simulink model "PC_Quadcopter_Simulation_Hexacopter_health"  (R2022b)
settings: Solver=ode4  StartTime=0.0  StopTime=100  FixedStep=0.01  MaxStep=0.06  RelTol=1e-3
PreLoadFcn:
  | DoB_parameter
model workspace (MAT data in the model file):
  Sig : Simulink.Signal (value not decoded)
values from neighbouring files (symbols this model uses):
  A = [ ... (first row only)    [DoB_parameter.m]
  B = [0 1 0]'    [DoB_parameter.m]
  C = [1 0 0]    [DoB_parameter.m]
  den_Inv_X = conv(num_X,den_Qfilter)    [DoB_parameter.m]
  den_Inv_Y = conv(num_Y, den_Qfilter)    [DoB_parameter.m]
  den_Inv_Z = conv(num_Z, den_Qfilter_Z)    [DoB_parameter.m]
  den_Qfilter = [1 a1/tau a0/tau^2]    [DoB_parameter.m]
  den_Qfilter_Z = [1 a1/tau a0/tau^2]    [DoB_parameter.m]
  I_xx = J(1,1)    [DoB_parameter.m]
  I_yy = J(2,2)    [DoB_parameter.m]
  I_zz = J(3,3)    [DoB_parameter.m]
  IC = block.DialogPrm(2).Data    [quadcopterDynamicsSFunction.m]
  L = [l1 l2 l3]'    [DoB_parameter.m]
  num_Inv_X = conv(den_X,num_Qfilter)    [DoB_parameter.m]
  num_Inv_Y = conv(den_Y, num_Qfilter)    [DoB_parameter.m]
  num_Inv_Z = conv(den_Z, num_Qfilter_Z)    [DoB_parameter.m]
  num_Qfilter = a0/tau^2    (= 100)    [DoB_parameter.m]
  num_Qfilter_Z = a0/tau^2    (= 11.1111111111)    [DoB_parameter.m]
undefined symbols (not defined in the file or in its folder): magnitude, quadModel
libraries: simulink x25, sharedTrackingLibrary x1
(part 2 of 2)

== system PC_Quadcopter_Simulation_Hexacopter_health/Fault Diagnosis/Generate Residual ==
  yMeasured[k] : Inport
  xEstimated[k|k] : Inport  Port=2
  RPM command : Inport  Port=3
  MATLAB Function - Generate Predicted Output : MATLAB Function  TreatAsAtomicUnit=on
  Subtract : Sum  Inputs=+-
  Unit Delay : UnitDelay  InitialCondition=zeros(15,1)  SampleTime=-1  HasFrameUpgradeWarning=on
  Residual : Outport
  wires:
  xEstimated[k|k]/1 -> Unit Delay/1
  Unit Delay/1 -> MATLAB Function - Generate Predicted Output/1(xEstimated)  "xEstimated[k-1|k-1]"
  MATLAB Function - Generate Predicted Output/1(yPredicted) -> Subtract/2  "yPredicted[k|k-1]"
  Subtract/1 -> Residual/1  "e[k]"
  yMeasured[k]/1 -> Subtract/1
  RPM command/1 -> MATLAB Function - Generate Predicted Output/2(u)

== system PC_Quadcopter_Simulation_Hexacopter_health/Hexacopter Dynamics/External Disturbances ==
  note: Note: Torques are in units of N*m, Forces in N
      | Torques are applied to the BODY coordinate system.
      | Forces are applied from the WORLD coordinate system!
      | This can be changed by adjusting the equations within the S-function.
  Bus Creator : BusCreator  Inputs=6
  Bus to Vector : BusToVector
  Constant{1..2,5..6} (4 alike) : Constant  Value=0
  Manual Switch : ManualSwitch
  Manual Switch1 : ManualSwitch
  Step : Step  Time=5  After=0.1  SampleTime=0
  Step2 : Step  Time=10  After=3  SampleTime=0
  "Disturbances " : Outport
  wires:
  Bus to Vector/1 -> "Disturbances "/1
  Bus Creator/1 -> Bus to Vector/1
  Constant6/1 -> Manual Switch1/1, Bus Creator/1  "Tau_bx-axis"
  Constant2/1 -> Bus Creator/3  "Tau_bz-axis"
  Constant1/1 -> Manual Switch/1, Bus Creator/4  "Force_x-axis"
  Constant5/1 -> Bus Creator/6  "Force_z-axis"
  Manual Switch/1 -> Bus Creator/5
  Step2/1 -> Manual Switch/2  "Force_y-axis"
  Manual Switch1/1 -> Bus Creator/2
  Step/1 -> Manual Switch1/2  "Tau_by-axis"

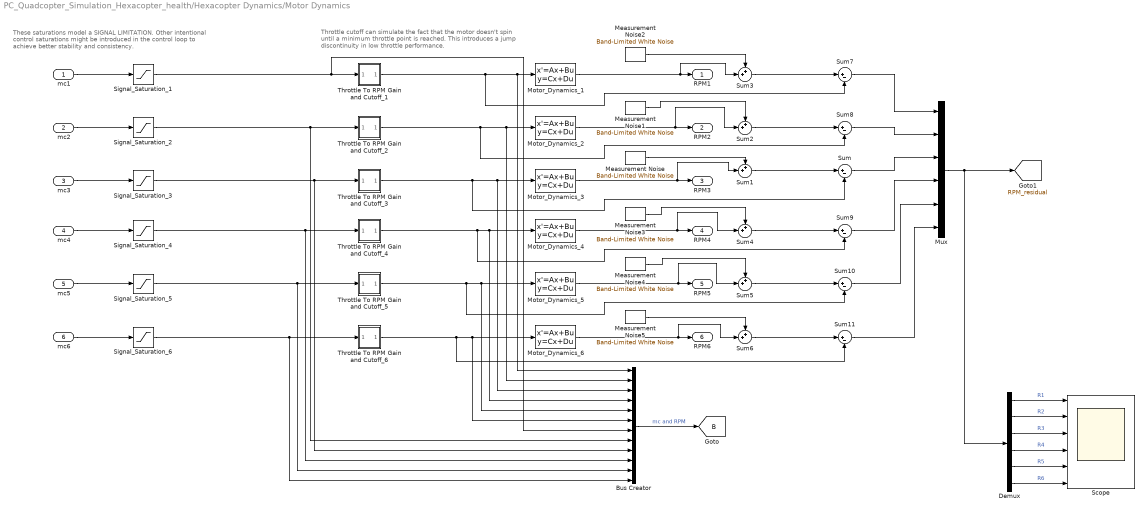
== system PC_Quadcopter_Simulation_Hexacopter_health/Hexacopter Dynamics/Motor Dynamics ==
  note: Throttle cutoff can simulate the fact that the motor doesn't
      | spin until a minimum throttle point is reached. This introduces
      | a jump discontinuity in low throttle performance.
  note: These saturations model a SIGNAL LIMITATION.
      | Other intentional control saturations might be introduced in the
      | control loop to achieve better stability and consistency.
  mc1 : Inport
  mc2 : Inport  Port=2
  mc3 : Inport  Port=3
  mc4 : Inport  Port=4
  mc5 : Inport  Port=5
  mc6 : Inport  Port=6
  Bus Creator : BusCreator  Inputs=12
  Demux : Demux  Outputs=6
  Measurement Noise{,1..5} (6 alike) : simulink/Sources/Band-Limited White Noise  Cov=10^2  Ts=0.02  seed=[23342]
  Motor_Dynamics_1 : StateSpace  A=-1/quadModel.T  C=1/quadModel.T  D=0  InitialCondition=IC.w1*quadModel.T
  Motor_Dynamics_2 : StateSpace  A=-1/quadModel.T  C=1/quadModel.T  D=0  InitialCondition=IC.w2*quadModel.T
  Motor_Dynamics_3 : StateSpace  A=-1/quadModel.T  C=1/quadModel.T  D=0  InitialCondition=IC.w3*quadModel.T
  Motor_Dynamics_4 : StateSpace  A=-1/quadModel.T  C=1/quadModel.T  D=0  InitialCondition=IC.w4*quadModel.T
  Motor_Dynamics_5 : StateSpace  A=-1/quadModel.T  C=1/quadModel.T  D=0  InitialCondition=IC.w4*quadModel.T
  Motor_Dynamics_6 : StateSpace  A=-1/quadModel.T  C=1/quadModel.T  D=0  InitialCondition=IC.w4*quadModel.T
  Mux : Mux  Inputs=6
  Scope : Scope  NumInputPorts=6
  Signal_Saturation_{1..6} (6 alike) : Saturate  UpperLimit=100  LowerLimit=0
  Sum{,7..11} (6 alike) : Sum  Inputs=|+-
  Sum{1..6} (6 alike) : Sum  Inputs=++|
  Throttle To RPM Gain and Cutoff_1 : Subsystem
  Throttle To RPM Gain and Cutoff_2 : Subsystem
  Throttle To RPM Gain and Cutoff_3 : Subsystem
  Throttle To RPM Gain and Cutoff_4 : Subsystem
  Throttle To RPM Gain and Cutoff_5 : Subsystem
  Throttle To RPM Gain and Cutoff_6 : Subsystem
  RPM1 : Outport
  RPM2 : Outport  Port=2
  RPM3 : Outport  Port=3
  RPM4 : Outport  Port=4
  RPM5 : Outport  Port=5
  RPM6 : Outport  Port=6
  tag scope: B=global, RPM_residual=global
  wires:
  mc1/1 -> Signal_Saturation_1/1
  mc4/1 -> Signal_Saturation_4/1
  mc2/1 -> Signal_Saturation_2/1
  mc3/1 -> Signal_Saturation_3/1
  Signal_Saturation_1/1 -> Bus Creator/7, Throttle To RPM Gain and Cutoff_1/1(In5)
  Signal_Saturation_2/1 -> Throttle To RPM Gain and Cutoff_2/1(In5), Bus Creator/8
  Signal_Saturation_3/1 -> Bus Creator/9, Throttle To RPM Gain and Cutoff_3/1(In5)
  Signal_Saturation_4/1 -> Bus Creator/10, Throttle To RPM Gain and Cutoff_4/1(In5)
  Throttle To RPM Gain and Cutoff_1/1(Out5) -> Sum7/2, Bus Creator/1, Motor_Dynamics_1/1
  Throttle To RPM Gain and Cutoff_2/1(Out5) -> Sum8/2, Motor_Dynamics_2/1, Bus Creator/2
  Throttle To RPM Gain and Cutoff_3/1(Out5) -> Sum/2, Motor_Dynamics_3/1, Bus Creator/3
  Throttle To RPM Gain and Cutoff_4/1(Out5) -> Sum9/2, Motor_Dynamics_4/1, Bus Creator/4
  Motor_Dynamics_1/1 -> Sum3/2, RPM1/1
  Motor_Dynamics_2/1 -> Sum2/2, RPM2/1
  Motor_Dynamics_3/1 -> Sum1/2, RPM3/1
  Motor_Dynamics_4/1 -> Sum4/2, RPM4/1
  Bus Creator/1 -> [B]  "mc and RPM"
  Motor_Dynamics_5/1 -> Sum5/2, RPM5/1
  mc5/1 -> Signal_Saturation_5/1
  Signal_Saturation_5/1 -> Bus Creator/11, Throttle To RPM Gain and Cutoff_5/1(In5)
  Throttle To RPM Gain and Cutoff_5/1(Out5) -> Sum10/2, Motor_Dynamics_5/1, Bus Creator/5
  Motor_Dynamics_6/1 -> Sum6/2, RPM6/1
  mc6/1 -> Signal_Saturation_6/1
  Signal_Saturation_6/1 -> Bus Creator/12, Throttle To RPM Gain and Cutoff_6/1(In5)
  Throttle To RPM Gain and Cutoff_6/1(Out5) -> Sum11/2, Motor_Dynamics_6/1, Bus Creator/6
  Mux/1 -> Demux/1, [RPM_residual]
  Measurement Noise/1 -> Sum1/1
  Sum1/1 -> Sum/1
  Measurement Noise5/1 -> Sum6/1
  Measurement Noise4/1 -> Sum5/1
  Measurement Noise3/1 -> Sum4/1
  Measurement Noise1/1 -> Sum2/1
  Measurement Noise2/1 -> Sum3/1
  Sum2/1 -> Sum8/1
  Sum3/1 -> Sum7/1
  Sum4/1 -> Sum9/1
  Sum5/1 -> Sum10/1
  Sum6/1 -> Sum11/1
  Sum7/1 -> Mux/1
  Sum8/1 -> Mux/2
  Sum/1 -> Mux/3
  Sum9/1 -> Mux/4
  Sum10/1 -> Mux/5
  Sum11/1 -> Mux/6
  Demux/6 -> Scope/6  "R6"
  Demux/5 -> Scope/5  "R5"
  Demux/4 -> Scope/4  "R4"
  Demux/3 -> Scope/3  "R3"
  Demux/2 -> Scope/2  "R2"
  Demux/1 -> Scope/1  "R1"

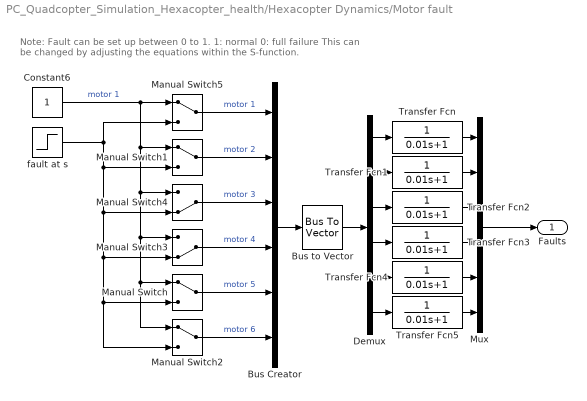
== system PC_Quadcopter_Simulation_Hexacopter_health/Hexacopter Dynamics/Motor fault ==
  note: Note: Fault can be set up between 0 to 1.
      | 1: normal
      | 0: full failure
      | This can be changed by adjusting the equations within the S-function.
  Bus Creator : BusCreator  Inputs=6
  Bus to Vector : BusToVector
  Constant6 : Constant
  Demux : Demux  Outputs=6
  Manual Switch{,1..2,5} (4 alike) : ManualSwitch
  Manual Switch3 : ManualSwitch  CurrentSetting=0
  Manual Switch4 : ManualSwitch  CurrentSetting=0
  Mux : Mux  Inputs=6
  Transfer Fcn{,1..5} (6 alike) : TransferFcn  Numerator=1  Denominator=[0.01 1]
  fault at s : Step  Time=85  Before=1  After=0  SampleTime=0
  Faults : Outport
  wires:
  Manual Switch1/1 -> Bus Creator/2  "motor 2"
  Manual Switch/1 -> Bus Creator/5  "motor 5"
  Bus Creator/1 -> Bus to Vector/1
  Manual Switch2/1 -> Bus Creator/6  "motor 6"
  Manual Switch3/1 -> Bus Creator/4  "motor 4"
  Demux/1 -> Transfer Fcn/1
  Demux/2 -> Transfer Fcn1/1
  Demux/3 -> Transfer Fcn2/1
  Demux/6 -> Transfer Fcn5/1
  Demux/5 -> Transfer Fcn4/1
  Demux/4 -> Transfer Fcn3/1
  Transfer Fcn/1 -> Mux/1
  Transfer Fcn1/1 -> Mux/2
  Transfer Fcn2/1 -> Mux/3
  Transfer Fcn4/1 -> Mux/5
  Transfer Fcn5/1 -> Mux/6
  Transfer Fcn3/1 -> Mux/4
  Manual Switch4/1 -> Bus Creator/3  "motor 3"
  Constant6/1 -> Manual Switch5/1, Manual Switch2/1, Manual Switch/1, Manual Switch3/1, Manual Switch4/1, Manual Switch1/1  "motor 1"
  Manual Switch5/1 -> Bus Creator/1  "motor 1"
  fault at s/1 -> Manual Switch2/2, Manual Switch/2, Manual Switch3/2, Manual Switch4/2, Manual Switch1/2, Manual Switch5/2
  Bus to Vector/1 -> Demux/1
  Mux/1 -> Faults/1

== system PC_Quadcopter_Simulation_Hexacopter_health/Hexacopter Dynamics/a_x, a_y, a_z ==
  p : Inport
  q : Inport  Port=2
  r : Inport  Port=3
  U : Inport  Port=4
  V : Inport  Port=5
  W : Inport  Port=6
  Phi : Inport  Port=7
  Theta : Inport  Port=8
  Subsystem : Subsystem
  Subsystem1 : Subsystem
  Subsystem2 : Subsystem
  a_x : Outport
  a_y : Outport  Port=2
  a_z : Outport  Port=3
  wires:
  Subsystem/1(a_x) -> a_x/1
  Subsystem1/1(a_y) -> a_y/1
  Subsystem2/1(a_z) -> a_z/1
  q/1 -> Subsystem2/2(q), Subsystem/1(q)
  r/1 -> Subsystem/2(r), Subsystem1/2(r)
  U/1 -> Subsystem2/3(U), Subsystem1/3(U), Subsystem/3(U)
  V/1 -> Subsystem2/4(V), Subsystem/4(V), Subsystem1/4(V)
  W/1 -> Subsystem2/5(W), Subsystem/5(W), Subsystem1/5(W)
  Theta/1 -> Subsystem2/7(Theta), Subsystem1/7(Theta), Subsystem/6(Theta)
  p/1 -> Subsystem2/1(p), Subsystem1/1(p)
  Phi/1 -> Subsystem2/6(Phi), Subsystem1/6(Phi)

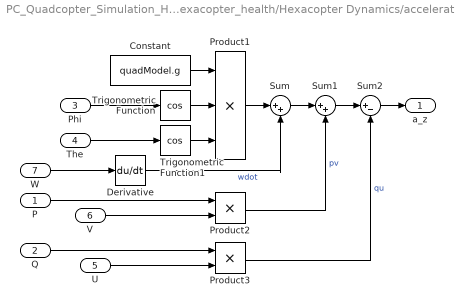
== system PC_Quadcopter_Simulation_Hexacopter_health/Hexacopter Dynamics/acceleration ==
  P : Inport
  Q : Inport  Port=2
  Phi : Inport  Port=3
  The : Inport  Port=4
  U : Inport  Port=5
  V : Inport  Port=6
  W : Inport  Port=7
  Constant : Constant  Value=quadModel.g
  Derivative : Derivative
  Product1 : Product  Inputs=3
  Product2 : Product
  Product3 : Product
  Sum : Sum  Inputs=|++
  Sum1 : Sum  Inputs=|++
  Sum2 : Sum  Inputs=|+-
  Trigonometric Function : Trigonometry  Operator=cos
  Trigonometric Function1 : Trigonometry  Operator=cos
  a_z : Outport
  wires:
  Trigonometric Function/1 -> Product1/2
  Sum/1 -> Sum1/1
  Derivative/1 -> Sum/2  "wdot"
  Trigonometric Function1/1 -> Product1/3
  W/1 -> Derivative/1
  Constant/1 -> Product1/1
  Sum1/1 -> Sum2/1
  Phi/1 -> Trigonometric Function/1
  V/1 -> Product2/2
  P/1 -> Product2/1
  U/1 -> Product3/2
  Sum2/1 -> a_z/1
  The/1 -> Trigonometric Function1/1
  Q/1 -> Product3/1
  Product2/1 -> Sum1/2  "pv"
  Product3/1 -> Sum2/2  "qu"
  Product1/1 -> Sum/1

== system PC_Quadcopter_Simulation_Hexacopter_health/LESO/Linear Extended-State Observer ==
  y : Inport
  u : Inport  Port=2
  Add3 : Sum  Inputs=+++
  Demux : Demux  Outputs=3
  Integrator : Integrator
  Terminator : Terminator
  theta1 : Gain  Gain=B  Multiplication=Matrix(K*u)
  theta10 : Gain  Gain=L  Multiplication=Matrix(K*u)
  theta2 : Gain  Gain=A-L*C  Multiplication=Matrix(K*u)
  x2_hat : Outport
  x3_hat (F) : Outport  Port=2
  wires:
  theta1/1 -> Add3/2
  theta10/1 -> Add3/1
  y/1 -> theta10/1
  u/1 -> theta1/1
  Add3/1 -> Integrator/1
  theta2/1 -> Add3/3
  Demux/3 -> x3_hat (F)/1
  Demux/2 -> x2_hat/1
  Integrator/1 -> theta2/1, Demux/1
  Demux/1 -> Terminator/1

== system PC_Quadcopter_Simulation_Hexacopter_health/LESO/Linear Extended-State Observer1 ==
  y : Inport
  u : Inport  Port=2
  Add3 : Sum  Commented=on  Inputs=+++
  Demux : Demux  Commented=on  Outputs=3
  Integrator : Integrator  Commented=on
  Terminator : Terminator  Commented=on
  theta1 : Gain  Commented=on  Gain=B  Multiplication=Matrix(K*u)
  theta10 : Gain  Commented=on  Gain=L  Multiplication=Matrix(K*u)
  theta2 : Gain  Commented=on  Gain=A-L*C  Multiplication=Matrix(K*u)
  x2_hat : Outport
  x3_hat (F) : Outport  Port=2
  wires:
  Demux/1 -> Terminator/1
  Integrator/1 -> Demux/1, theta2/1
  Demux/2 -> x2_hat/1
  Demux/3 -> x3_hat (F)/1
  theta2/1 -> Add3/3
  Add3/1 -> Integrator/1
  u/1 -> theta1/1
  y/1 -> theta10/1
  theta10/1 -> Add3/1
  theta1/1 -> Add3/2

== system PC_Quadcopter_Simulation_Hexacopter_health/LESO/Linear Extended-State Observer2 ==
  y : Inport
  u : Inport  Port=2
  Add3 : Sum  Inputs=+++
  Demux : Demux  Outputs=3
  Integrator : Integrator
  Terminator : Terminator
  theta1 : Gain  Gain=B  Multiplication=Matrix(K*u)
  theta10 : Gain  Gain=L  Multiplication=Matrix(K*u)
  theta2 : Gain  Gain=A-L*C  Multiplication=Matrix(K*u)
  x2_hat : Outport
  x3_hat (F) : Outport  Port=2
  wires:
  theta1/1 -> Add3/2
  theta10/1 -> Add3/1
  y/1 -> theta10/1
  u/1 -> theta1/1
  Add3/1 -> Integrator/1
  theta2/1 -> Add3/3
  Demux/3 -> x3_hat (F)/1
  Demux/2 -> x2_hat/1
  Integrator/1 -> theta2/1, Demux/1
  Demux/1 -> Terminator/1

== system PC_Quadcopter_Simulation_Hexacopter_health/Position Controller/Altitude (Z) Control ==
  note: Improve to use rotation matrix and euler angles...
      | maybe with saturation?
  note: ez
  Desired Z : Inport
  Bus Selector : BusSelector  OutputSignals=Alt_Cmd
  Gravity Offset (Level Flight) : Constant  Value=GOffset
  Integrator Limited : Integrator  LimitOutput=on  UpperSaturationLimit=USat  LowerSaturationLimit=LSat
  Kiz : Gain  Gain=Kiz
  Kpz : Gain  Gain=Kpz
  Sum : Sum  Inputs=|+|
  Sum2 : Sum  Inputs=+++
  Alt. (Z) Correction : Outport
  wires:
  Gravity Offset (Level Flight)/1 -> Sum2/1
  Desired Z/1 -> Bus Selector/1
  Sum2/1 -> Alt. (Z) Correction/1
  Kpz/1 -> Sum2/2  "P Corr"
  Sum/1 -> Integrator Limited/1, Kpz/1  "Error"
  Kiz/1 -> Sum2/3  "I Corr"
  Integrator Limited/1 -> Kiz/1
  Bus Selector/1 -> Sum/1  "<Alt_Cmd>"

== system PC_Quadcopter_Simulation_Hexacopter_health/Position Controller/Error Rotations ==
  X_cmd : Inport
  Y_cmd : Inport  Port=2
  X : Inport  Port=3
  Y : Inport  Port=4
  Psi : Inport  Port=5
  Product{,1..3} (4 alike) : Product
  Sum : Sum  Inputs=|+-
  Sum1 : Sum  Inputs=|+-
  Sum2 : Sum  Inputs=|++
  Sum4 : Sum  Inputs=|+-
  Trigonometric Functions : Trigonometry  Operator=sincos
  X Error in body Frame : Outport
  Y Error in Body Frame : Outport  Port=2
  wires:
  Sum4/1 -> Y Error in Body Frame/1  "Yerr*cos(psi)-Xerr*sin(psi)"
  Product3/1 -> Sum4/2  "Xerr*sin(psi)"
  Sum1/1 -> Product2/1, Product1/1  "Y Error"
  Trigonometric Functions/1 -> Product2/2, Product3/2  "sin(psi)"
  Sum2/1 -> X Error in body Frame/1  "Xerr*cos(psi)+Yerr*sin(psi)"
  Y_cmd/1 -> Sum1/1
  X_cmd/1 -> Sum/1
  X/1 -> Sum/2
  Y/1 -> Sum1/2
  Sum/1 -> Product3/1, Product/1  "X Error"
  Trigonometric Functions/2 -> Product/2, Product1/2  "cos(psi)"
  Product/1 -> Sum2/1  "Xerr*cos(psi)"
  Product2/1 -> Sum2/2  "Yerr*sin(psi)"
  Product1/1 -> Sum4/1  "Yerr*cos(psi)"
  Psi/1 -> Trigonometric Functions/1

== system PC_Quadcopter_Simulation_Hexacopter_health/Position Controller/Error Rotations1 ==
  X_cmd : Inport
  Y_cmd : Inport  Port=2
  Constant : Constant  Value=0
  Product{,1..3} (4 alike) : Product
  Sum2 : Sum  Inputs=|++
  Sum4 : Sum  Inputs=|+-
  Trigonometric Functions : Trigonometry  Operator=sincos
  X Error in body Frame : Outport
  Y Error in Body Frame : Outport  Port=2
  wires:
  Constant/1 -> Trigonometric Functions/1
  Product1/1 -> Sum4/1  "Yerr*cos(psi)"
  Product2/1 -> Sum2/2  "Yerr*sin(psi)"
  Product/1 -> Sum2/1  "Xerr*cos(psi)"
  Trigonometric Functions/2 -> Product1/2, Product/2  "cos(psi)"
  X_cmd/1 -> Product/1, Product3/1  "X Error"
  Sum2/1 -> X Error in body Frame/1  "Xerr*cos(psi)+Yerr*sin(psi)"
  Trigonometric Functions/1 -> Product3/2, Product2/2  "sin(psi)"
  Y_cmd/1 -> Product1/1, Product2/1  "Y Error"
  Product3/1 -> Sum4/2  "Xerr*sin(psi)"
  Sum4/1 -> Y Error in Body Frame/1  "Yerr*cos(psi)-Xerr*sin(psi)"

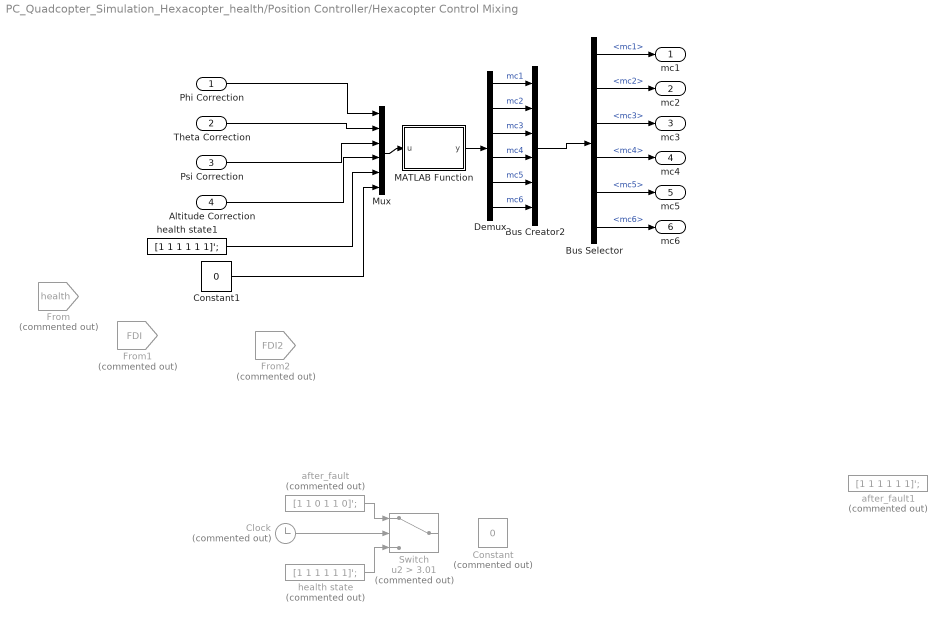
== system PC_Quadcopter_Simulation_Hexacopter_health/Position Controller/Hexacopter Control Mixing ==
  Phi Correction : Inport
  Theta Correction : Inport  Port=2
  Psi Correction : Inport  Port=3
  Altitude Correction : Inport  Port=4
  Bus Creator2 : BusCreator  Inputs=6
  Bus Selector : BusSelector  OutputSignals=mc1,mc2,mc3,mc4,mc5,mc6
  Clock : Clock  Commented=on
  Constant : Constant  Commented=on  Value=0
  Constant1 : Constant  Value=0
  Demux : Demux  Outputs=6
  From : From  Commented=on  GotoTag=health  TagVisibility=global
  From1 : From  Commented=on  GotoTag=FDI  TagVisibility=global
  From2 : From  Commented=on  GotoTag=FDI2  TagVisibility=global
  MATLAB Function : MATLAB Function  TreatAsAtomicUnit=on
  Mux : Mux  Inputs=6
  Switch : Switch  Commented=on  Criteria=u2 > Threshold  Threshold=3.01  SaturateOnIntegerOverflow=off  InputSameDT=off
  after_fault : Constant  Commented=on  Value=[1 1 0 1 1 0]';
  after_fault1 : Constant  Commented=on  Value=[1 1 1 1 1 1]';
  health state : Constant  Commented=on  Value=[1 1 1 1 1 1]';
  health state1 : Constant  Value=[1 1 1 1 1 1]';
  mc1 : Outport
  mc2 : Outport  Port=2
  mc3 : Outport  Port=3
  mc4 : Outport  Port=4
  mc5 : Outport  Port=5
  mc6 : Outport  Port=6
  wires:
  Phi Correction/1 -> Mux/1
  Theta Correction/1 -> Mux/2
  Psi Correction/1 -> Mux/3
  Altitude Correction/1 -> Mux/4
  Bus Selector/1 -> mc1/1  "<mc1>"
  Bus Selector/2 -> mc2/1  "<mc2>"
  Bus Selector/3 -> mc3/1  "<mc3>"
  Bus Selector/4 -> mc4/1  "<mc4>"
  Bus Selector/5 -> mc5/1  "<mc5>"
  Bus Selector/6 -> mc6/1  "<mc6>"
  Mux/1 -> MATLAB Function/1(u)
  MATLAB Function/1(y) -> Demux/1
  Demux/6 -> Bus Creator2/6  "mc6"
  Demux/3 -> Bus Creator2/3  "mc3"
  Demux/4 -> Bus Creator2/4  "mc4"
  Demux/1 -> Bus Creator2/1  "mc1"
  Demux/5 -> Bus Creator2/5  "mc5"
  Demux/2 -> Bus Creator2/2  "mc2"
  Bus Creator2/1 -> Bus Selector/1
  Constant1/1 -> Mux/6
  health state1/1 -> Mux/5
  health state/1 -> Switch/3
  after_fault/1 -> Switch/1
  Clock/1 -> Switch/2

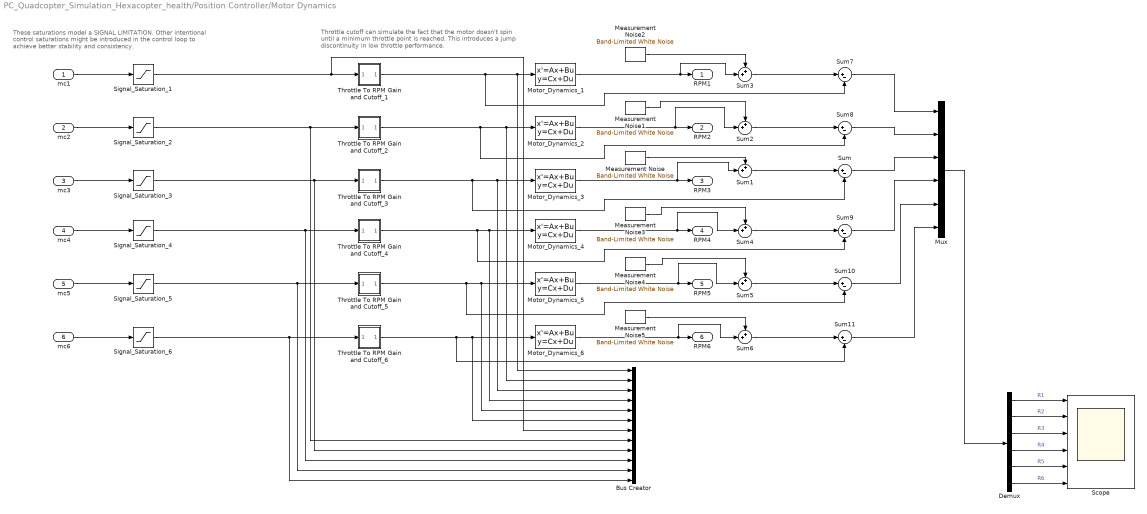
== system PC_Quadcopter_Simulation_Hexacopter_health/Position Controller/Motor Dynamics ==
  note: Throttle cutoff can simulate the fact that the motor doesn't
      | spin until a minimum throttle point is reached. This introduces
      | a jump discontinuity in low throttle performance.
  note: These saturations model a SIGNAL LIMITATION.
      | Other intentional control saturations might be introduced in the
      | control loop to achieve better stability and consistency.
  mc1 : Inport
  mc2 : Inport  Port=2
  mc3 : Inport  Port=3
  mc4 : Inport  Port=4
  mc5 : Inport  Port=5
  mc6 : Inport  Port=6
  Bus Creator : BusCreator  Inputs=12
  Demux : Demux  Outputs=6
  Measurement Noise{,1..5} (6 alike) : simulink/Sources/Band-Limited White Noise  Cov=10^2  Ts=0.02  seed=[23342]
  Motor_Dynamics_1 : StateSpace  A=-1/quadModel.T  C=1/quadModel.T  D=0  InitialCondition=IC.w1*quadModel.T
  Motor_Dynamics_2 : StateSpace  A=-1/quadModel.T  C=1/quadModel.T  D=0  InitialCondition=IC.w2*quadModel.T
  Motor_Dynamics_3 : StateSpace  A=-1/quadModel.T  C=1/quadModel.T  D=0  InitialCondition=IC.w3*quadModel.T
  Motor_Dynamics_4 : StateSpace  A=-1/quadModel.T  C=1/quadModel.T  D=0  InitialCondition=IC.w4*quadModel.T
  Motor_Dynamics_5 : StateSpace  A=-1/quadModel.T  C=1/quadModel.T  D=0  InitialCondition=IC.w4*quadModel.T
  Motor_Dynamics_6 : StateSpace  A=-1/quadModel.T  C=1/quadModel.T  D=0  InitialCondition=IC.w4*quadModel.T
  Mux : Mux  Inputs=6
  Scope : Scope  NumInputPorts=6
  Signal_Saturation_{1..6} (6 alike) : Saturate  UpperLimit=100  LowerLimit=0
  Sum{,7..11} (6 alike) : Sum  Inputs=|+-
  Sum{1..6} (6 alike) : Sum  Inputs=++|
  Throttle To RPM Gain and Cutoff_1 : Subsystem
  Throttle To RPM Gain and Cutoff_2 : Subsystem
  Throttle To RPM Gain and Cutoff_3 : Subsystem
  Throttle To RPM Gain and Cutoff_4 : Subsystem
  Throttle To RPM Gain and Cutoff_5 : Subsystem
  Throttle To RPM Gain and Cutoff_6 : Subsystem
  RPM1 : Outport
  RPM2 : Outport  Port=2
  RPM3 : Outport  Port=3
  RPM4 : Outport  Port=4
  RPM5 : Outport  Port=5
  RPM6 : Outport  Port=6
  wires:
  mc1/1 -> Signal_Saturation_1/1
  mc4/1 -> Signal_Saturation_4/1
  mc2/1 -> Signal_Saturation_2/1
  mc3/1 -> Signal_Saturation_3/1
  Signal_Saturation_1/1 -> Bus Creator/7, Throttle To RPM Gain and Cutoff_1/1(In5)
  Signal_Saturation_2/1 -> Throttle To RPM Gain and Cutoff_2/1(In5), Bus Creator/8
  Signal_Saturation_3/1 -> Bus Creator/9, Throttle To RPM Gain and Cutoff_3/1(In5)
  Signal_Saturation_4/1 -> Bus Creator/10, Throttle To RPM Gain and Cutoff_4/1(In5)
  Throttle To RPM Gain and Cutoff_1/1(Out5) -> Sum7/2, Bus Creator/1, Motor_Dynamics_1/1
  Throttle To RPM Gain and Cutoff_2/1(Out5) -> Sum8/2, Motor_Dynamics_2/1, Bus Creator/2
  Throttle To RPM Gain and Cutoff_3/1(Out5) -> Sum/2, Motor_Dynamics_3/1, Bus Creator/3
  Throttle To RPM Gain and Cutoff_4/1(Out5) -> Sum9/2, Motor_Dynamics_4/1, Bus Creator/4
  Motor_Dynamics_1/1 -> Sum3/2, RPM1/1
  Motor_Dynamics_2/1 -> Sum2/2, RPM2/1
  Motor_Dynamics_3/1 -> Sum1/2, RPM3/1
  Motor_Dynamics_4/1 -> Sum4/2, RPM4/1
  Motor_Dynamics_5/1 -> Sum5/2, RPM5/1
  mc5/1 -> Signal_Saturation_5/1
  Signal_Saturation_5/1 -> Bus Creator/11, Throttle To RPM Gain and Cutoff_5/1(In5)
  Throttle To RPM Gain and Cutoff_5/1(Out5) -> Sum10/2, Motor_Dynamics_5/1, Bus Creator/5
  Motor_Dynamics_6/1 -> Sum6/2, RPM6/1
  mc6/1 -> Signal_Saturation_6/1
  Signal_Saturation_6/1 -> Bus Creator/12, Throttle To RPM Gain and Cutoff_6/1(In5)
  Throttle To RPM Gain and Cutoff_6/1(Out5) -> Sum11/2, Motor_Dynamics_6/1, Bus Creator/6
  Mux/1 -> Demux/1
  Measurement Noise/1 -> Sum1/1
  Sum1/1 -> Sum/1
  Measurement Noise5/1 -> Sum6/1
  Measurement Noise4/1 -> Sum5/1
  Measurement Noise3/1 -> Sum4/1
  Measurement Noise1/1 -> Sum2/1
  Measurement Noise2/1 -> Sum3/1
  Sum2/1 -> Sum8/1
  Sum3/1 -> Sum7/1
  Sum4/1 -> Sum9/1
  Sum5/1 -> Sum10/1
  Sum6/1 -> Sum11/1
  Sum7/1 -> Mux/1
  Sum8/1 -> Mux/2
  Sum/1 -> Mux/3
  Sum9/1 -> Mux/4
  Sum10/1 -> Mux/5
  Sum11/1 -> Mux/6
  Demux/6 -> Scope/6  "R6"
  Demux/5 -> Scope/5  "R5"
  Demux/4 -> Scope/4  "R4"
  Demux/3 -> Scope/3  "R3"
  Demux/2 -> Scope/2  "R2"
  Demux/1 -> Scope/1  "R1"

== system PC_Quadcopter_Simulation_Hexacopter_health/Position Controller/Phi Command Control ==
  note: -1 Gain is required because a "negative"
      | angle of Phi induces a positive velocity
      | in the body frame y direction!
  Desired Yb Velocity : Inport
  Yb Velocity : Inport  Port=2
  Attitude Limits_Phi : Saturate  UpperLimit=ASat  LowerLimit=-ASat
  Gain : Gain  Gain=-1
  Kdp : Gain  Gain=Kd
  Kpp : Gain  Gain=Kp
  Sum3 : Sum  Inputs=|+-
  Sum6 : Sum  Inputs=|+-
  V Derivative : Derivative
  Phi_cmd : Outport
  wires:
  V Derivative/1 -> Kdp/1
  Attitude Limits_Phi/1 -> Phi_cmd/1  "Phi_cmd"
  Sum6/1 -> Gain/1
  Kpp/1 -> Sum6/1
  Sum3/1 -> Kpp/1  "Velocity Error"
  Yb Velocity/1 -> V Derivative/1, Sum3/2
  Desired Yb Velocity/1 -> Sum3/1
  Gain/1 -> Attitude Limits_Phi/1
  Kdp/1 -> Sum6/2

== system PC_Quadcopter_Simulation_Hexacopter_health/Position Controller/Phi Command Control1 ==
  note: -1 Gain is required because a "negative"
      | angle of Phi induces a positive velocity
      | in the body frame y direction!
  Desired Yb Velocity : Inport
  Attitude Limits_Phi : Saturate  UpperLimit=ASat  LowerLimit=-ASat
  Gain : Gain  Gain=-1
  Kpp : Gain  Gain=Kp
  Phi_cmd : Outport
  wires:
  Gain/1 -> Attitude Limits_Phi/1
  Desired Yb Velocity/1 -> Kpp/1  "Velocity Error"
  Kpp/1 -> Gain/1
  Attitude Limits_Phi/1 -> Phi_cmd/1  "Phi_cmd"

== system PC_Quadcopter_Simulation_Hexacopter_health/Position Controller/Pitch (Theta) Control ==
  Attitude Command : Inport
  Bus Selector : BusSelector  OutputSignals=The_cmd
  Integrator Limited : Integrator  LimitOutput=on  UpperSaturationLimit=USat  LowerSaturationLimit=LSat
  Kit : Gain  Gain=Kit
  Kpt : Gain  Gain=Kpt
  Sum1 : Sum  Inputs=++|
  Theta Correction : Outport
  wires:
  Attitude Command/1 -> Bus Selector/1
  Sum1/1 -> Theta Correction/1
  Kpt/1 -> Sum1/1  "P Corr"
  Kit/1 -> Sum1/2  "I Corr"
  Integrator Limited/1 -> Kit/1
  Bus Selector/1 -> Integrator Limited/1, Kpt/1  "<The_cmd>"

== system PC_Quadcopter_Simulation_Hexacopter_health/Position Controller/Roll (Phi) Control  ==
  "Attitude Command " : Inport
  Bus Selector : BusSelector  OutputSignals=Phi_cmd
  Integrator Limited : Integrator  LimitOutput=on  UpperSaturationLimit=USat  LowerSaturationLimit=LSat
  Kip : Gain  Gain=Kip
  Kpp : Gain  Gain=Kpp
  Sum1 : Sum  Inputs=++|
  Phi Correction : Outport
  wires:
  Sum1/1 -> Phi Correction/1
  Kpp/1 -> Sum1/1  "P Corr"
  Kip/1 -> Sum1/2  "I Corr"
  Integrator Limited/1 -> Kip/1
  "Attitude Command "/1 -> Bus Selector/1
  Bus Selector/1 -> Integrator Limited/1, Kpp/1  "<Phi_cmd>"

== system PC_Quadcopter_Simulation_Hexacopter_health/Position Controller/Theta Command Control ==
  Desired Xb Velocity : Inport
  Xb Velocity : Inport  Port=2
  Attitude Limits_Theta : Saturate  UpperLimit=ASat  LowerLimit=-ASat
  Kdt : Gain  Gain=Kd
  Kpt : Gain  Gain=Kp
  Sum3 : Sum  Inputs=|+-
  Sum6 : Sum  Inputs=|+-
  U Derivative : Derivative
  The_cmd : Outport
  wires:
  Kdt/1 -> Sum6/2
  U Derivative/1 -> Kdt/1
  Attitude Limits_Theta/1 -> The_cmd/1  "The_cmd"
  Sum6/1 -> Attitude Limits_Theta/1
  Kpt/1 -> Sum6/1
  Sum3/1 -> Kpt/1  "Velocity Error"
  Xb Velocity/1 -> U Derivative/1, Sum3/2
  Desired Xb Velocity/1 -> Sum3/1

== system PC_Quadcopter_Simulation_Hexacopter_health/Position Controller/Theta Command Control1 ==
  Desired Xb Velocity : Inport
  Attitude Limits_Theta : Saturate  UpperLimit=ASat  LowerLimit=-ASat
  Kpt : Gain  Gain=Kp
  The_cmd : Outport
  wires:
  Desired Xb Velocity/1 -> Kpt/1  "Velocity Error"
  Kpt/1 -> Attitude Limits_Theta/1
  Attitude Limits_Theta/1 -> The_cmd/1  "The_cmd"

== system PC_Quadcopter_Simulation_Hexacopter_health/Position Controller/Yaw (Psi) Control ==
  Attitude Command : Inport
  Bus Selector : BusSelector  OutputSignals=Psi_cmd
  Integrator Limited : Integrator  LimitOutput=on  UpperSaturationLimit=USat  LowerSaturationLimit=LSat
  Kit : Gain  Gain=Kis
  Kps : Gain  Gain=Kps
  Sum1 : Sum  Inputs=++|
  Psi Correction : Outport
  wires:
  Attitude Command/1 -> Bus Selector/1
  Sum1/1 -> Psi Correction/1
  Kps/1 -> Sum1/1  "P Corr"
  Kit/1 -> Sum1/2  "I Corr"
  Integrator Limited/1 -> Kit/1
  Bus Selector/1 -> Integrator Limited/1, Kps/1  "<Psi_cmd>"

== system PC_Quadcopter_Simulation_Hexacopter_health/Hexacopter Dynamics/Motor Dynamics/Throttle To RPM Gain and Cutoff_1 ==
  note: minThr should be a quad.mat value
  note: This gain should be a quad.mat value
  note: This constant should be a quad.mat value
  note: Output equals linearly scaled RPM
      | for given throttle input if throttle input >=Throttle Cuttoff (minThr)
      | else output is zero.
  In5 : Inport
  Constant : Constant  Value=quadModel.b
  Gain : Gain  Gain=quadModel.cr
  Minimum Throttle Cutoff : simulink/Logic and Bit Operations/Compare To Constant  relop=>=  const=quadModel.minThr  OutDataTypeStr=uint8
  Product : Product
  Sum1 : Sum  Inputs=++|
  Out5 : Outport
  wires:
  Minimum Throttle Cutoff/1 -> Product/2
  Product/1 -> Out5/1
  In5/1 -> Gain/1, Minimum Throttle Cutoff/1
  Gain/1 -> Sum1/2
  Sum1/1 -> Product/1
  Constant/1 -> Sum1/1

== system PC_Quadcopter_Simulation_Hexacopter_health/Hexacopter Dynamics/Motor Dynamics/Throttle To RPM Gain and Cutoff_2 ==
  note: minThr should be a quad.mat value
  note: This gain should be a quad.mat value
  note: This constant should be a quad.mat value
  note: Output equals linearly scaled RPM
      | for given throttle input if throttle input >=Throttle Cuttoff (minThr)
      | else output is zero.
  In5 : Inport
  Constant : Constant  Value=quadModel.b
  Gain : Gain  Gain=quadModel.cr
  Minimum Throttle Cutoff : simulink/Logic and Bit Operations/Compare To Constant  relop=>=  const=quadModel.minThr  OutDataTypeStr=uint8
  Product : Product
  Sum1 : Sum  Inputs=++|
  Out5 : Outport
  wires:
  Minimum Throttle Cutoff/1 -> Product/2
  Product/1 -> Out5/1
  In5/1 -> Gain/1, Minimum Throttle Cutoff/1
  Gain/1 -> Sum1/2
  Sum1/1 -> Product/1
  Constant/1 -> Sum1/1

== system PC_Quadcopter_Simulation_Hexacopter_health/Hexacopter Dynamics/Motor Dynamics/Throttle To RPM Gain and Cutoff_3 ==
  note: minThr should be a quad.mat value
  note: This gain should be a quad.mat value
  note: This constant should be a quad.mat value
  note: Output equals linearly scaled RPM
      | for given throttle input if throttle input >=Throttle Cuttoff (minThr)
      | else output is zero.
  In5 : Inport
  Constant : Constant  Value=quadModel.b
  Gain : Gain  Gain=quadModel.cr
  Minimum Throttle Cutoff : simulink/Logic and Bit Operations/Compare To Constant  relop=>=  const=quadModel.minThr  OutDataTypeStr=uint8
  Product : Product
  Sum1 : Sum  Inputs=++|
  Out5 : Outport
  wires:
  Minimum Throttle Cutoff/1 -> Product/2
  Product/1 -> Out5/1
  In5/1 -> Gain/1, Minimum Throttle Cutoff/1
  Gain/1 -> Sum1/2
  Sum1/1 -> Product/1
  Constant/1 -> Sum1/1

== system PC_Quadcopter_Simulation_Hexacopter_health/Hexacopter Dynamics/Motor Dynamics/Throttle To RPM Gain and Cutoff_4 ==
  note: minThr should be a quad.mat value
  note: This gain should be a quad.mat value
  note: This constant should be a quad.mat value
  note: Output equals linearly scaled RPM
      | for given throttle input if throttle input >=Throttle Cuttoff (minThr)
      | else output is zero.
  In5 : Inport
  Constant : Constant  Value=quadModel.b
  Gain : Gain  Gain=quadModel.cr
  Minimum Throttle Cutoff : simulink/Logic and Bit Operations/Compare To Constant  relop=>=  const=quadModel.minThr  OutDataTypeStr=uint8
  Product : Product
  Sum1 : Sum  Inputs=++|
  Out5 : Outport
  wires:
  Minimum Throttle Cutoff/1 -> Product/2
  Product/1 -> Out5/1
  In5/1 -> Gain/1, Minimum Throttle Cutoff/1
  Gain/1 -> Sum1/2
  Sum1/1 -> Product/1
  Constant/1 -> Sum1/1

== system PC_Quadcopter_Simulation_Hexacopter_health/Hexacopter Dynamics/Motor Dynamics/Throttle To RPM Gain and Cutoff_5 ==
  note: minThr should be a quad.mat value
  note: This gain should be a quad.mat value
  note: This constant should be a quad.mat value
  note: Output equals linearly scaled RPM
      | for given throttle input if throttle input >=Throttle Cuttoff (minThr)
      | else output is zero.
  In5 : Inport
  Constant : Constant  Value=quadModel.b
  Gain : Gain  Gain=quadModel.cr
  Minimum Throttle Cutoff : simulink/Logic and Bit Operations/Compare To Constant  relop=>=  const=quadModel.minThr  OutDataTypeStr=uint8
  Product : Product
  Sum1 : Sum  Inputs=++|
  Out5 : Outport
  wires:
  Minimum Throttle Cutoff/1 -> Product/2
  Product/1 -> Out5/1
  In5/1 -> Gain/1, Minimum Throttle Cutoff/1
  Gain/1 -> Sum1/2
  Sum1/1 -> Product/1
  Constant/1 -> Sum1/1

== system PC_Quadcopter_Simulation_Hexacopter_health/Hexacopter Dynamics/Motor Dynamics/Throttle To RPM Gain and Cutoff_6 ==
  note: minThr should be a quad.mat value
  note: This gain should be a quad.mat value
  note: This constant should be a quad.mat value
  note: Output equals linearly scaled RPM
      | for given throttle input if throttle input >=Throttle Cuttoff (minThr)
      | else output is zero.
  In5 : Inport
  Constant : Constant  Value=quadModel.b
  Gain : Gain  Gain=quadModel.cr
  Minimum Throttle Cutoff : simulink/Logic and Bit Operations/Compare To Constant  relop=>=  const=quadModel.minThr  OutDataTypeStr=uint8
  Product : Product
  Sum1 : Sum  Inputs=++|
  Out5 : Outport
  wires:
  Minimum Throttle Cutoff/1 -> Product/2
  Product/1 -> Out5/1
  In5/1 -> Gain/1, Minimum Throttle Cutoff/1
  Gain/1 -> Sum1/2
  Sum1/1 -> Product/1
  Constant/1 -> Sum1/1

== system PC_Quadcopter_Simulation_Hexacopter_health/Hexacopter Dynamics/a_x, a_y, a_z/Subsystem ==
  q : Inport
  r : Inport  Port=2
  U : Inport  Port=3
  V : Inport  Port=4
  W : Inport  Port=5
  Theta : Inport  Port=6
  Constant : Constant  Value=quadModel.g
  Cos : Trigonometry
  Derivative : Derivative
  Product : Product
  Product1 : Product
  Product2 : Product
  Sum : Sum  Inputs=+--
  Sum1 : Sum  Inputs=|++
  a_x : Outport
  wires:
  Theta/1 -> Cos/1
  Cos/1 -> Product/1
  Constant/1 -> Product/2
  Product1/1 -> Sum1/1
  Derivative/1 -> Sum1/2
  Sum1/1 -> Sum/1
  Sum/1 -> a_x/1
  Product2/1 -> Sum/2
  Product/1 -> Sum/3
  U/1 -> Derivative/1
  q/1 -> Product1/1
  W/1 -> Product1/2
  r/1 -> Product2/1
  V/1 -> Product2/2

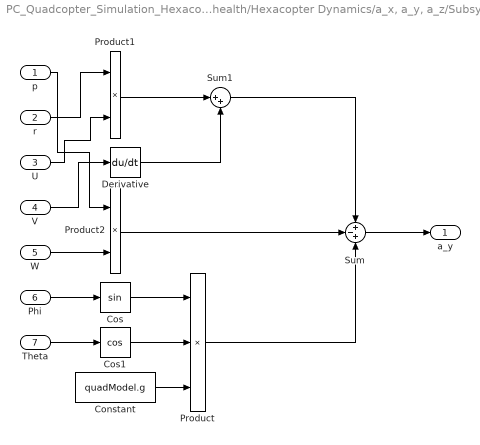
== system PC_Quadcopter_Simulation_Hexacopter_health/Hexacopter Dynamics/a_x, a_y, a_z/Subsystem1 ==
  p : Inport
  r : Inport  Port=2
  U : Inport  Port=3
  V : Inport  Port=4
  W : Inport  Port=5
  Phi : Inport  Port=6
  Theta : Inport  Port=7
  Constant : Constant  Value=quadModel.g
  Cos : Trigonometry
  Cos1 : Trigonometry  Operator=cos
  Derivative : Derivative
  Product : Product  Inputs=3
  Product1 : Product
  Product2 : Product
  Sum : Sum  Inputs=+-+
  Sum1 : Sum  Inputs=|++
  a_y : Outport
  wires:
  V/1 -> Derivative/1
  Theta/1 -> Cos1/1
  Phi/1 -> Cos/1
  Cos/1 -> Product/1
  Cos1/1 -> Product/2
  Constant/1 -> Product/3
  Derivative/1 -> Sum1/2
  r/1 -> Product1/1
  U/1 -> Product1/2
  W/1 -> Product2/2
  p/1 -> Product2/1
  Product1/1 -> Sum1/1
  Product2/1 -> Sum/2
  Sum1/1 -> Sum/1
  Product/1 -> Sum/3
  Sum/1 -> a_y/1

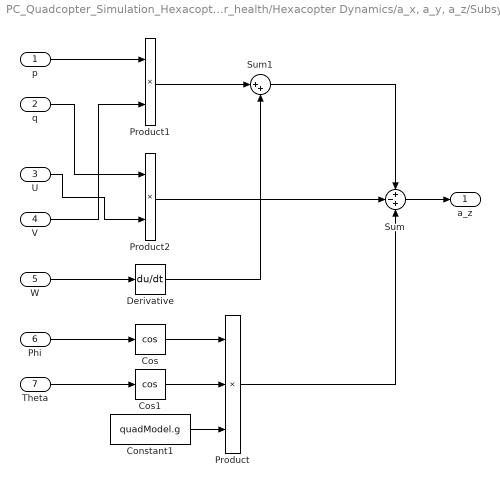
== system PC_Quadcopter_Simulation_Hexacopter_health/Hexacopter Dynamics/a_x, a_y, a_z/Subsystem2 ==
  p : Inport
  q : Inport  Port=2
  U : Inport  Port=3
  V : Inport  Port=4
  W : Inport  Port=5
  Phi : Inport  Port=6
  Theta : Inport  Port=7
  Constant1 : Constant  Value=quadModel.g
  Cos : Trigonometry  Operator=cos
  Cos1 : Trigonometry  Operator=cos
  Derivative : Derivative
  Product : Product  Inputs=3
  Product1 : Product
  Product2 : Product
  Sum : Sum  Inputs=+-+
  Sum1 : Sum  Inputs=|++
  a_z : Outport
  wires:
  Cos1/1 -> Product/2
  Constant1/1 -> Product/3
  Cos/1 -> Product/1
  Sum/1 -> a_z/1
  Theta/1 -> Cos1/1
  Phi/1 -> Cos/1
  W/1 -> Derivative/1
  p/1 -> Product1/1
  V/1 -> Product1/2
  q/1 -> Product2/1
  U/1 -> Product2/2
  Product1/1 -> Sum1/1
  Derivative/1 -> Sum1/2
  Product2/1 -> Sum/2
  Sum1/1 -> Sum/1
  Product/1 -> Sum/3

== system PC_Quadcopter_Simulation_Hexacopter_health/Position Controller/Motor Dynamics/Throttle To RPM Gain and Cutoff_1 ==
  note: minThr should be a quad.mat value
  note: This gain should be a quad.mat value
  note: This constant should be a quad.mat value
  note: Output equals linearly scaled RPM
      | for given throttle input if throttle input >=Throttle Cuttoff (minThr)
      | else output is zero.
  In5 : Inport
  Constant : Constant  Value=quadModel.b
  Gain : Gain  Gain=quadModel.cr
  Minimum Throttle Cutoff : simulink/Logic and Bit Operations/Compare To Constant  relop=>=  const=quadModel.minThr  OutDataTypeStr=uint8
  Product : Product
  Sum1 : Sum  Inputs=++|
  Out5 : Outport
  wires:
  Minimum Throttle Cutoff/1 -> Product/2
  Product/1 -> Out5/1
  In5/1 -> Gain/1, Minimum Throttle Cutoff/1
  Gain/1 -> Sum1/2
  Sum1/1 -> Product/1
  Constant/1 -> Sum1/1

== system PC_Quadcopter_Simulation_Hexacopter_health/Position Controller/Motor Dynamics/Throttle To RPM Gain and Cutoff_2 ==
  note: minThr should be a quad.mat value
  note: This gain should be a quad.mat value
  note: This constant should be a quad.mat value
  note: Output equals linearly scaled RPM
      | for given throttle input if throttle input >=Throttle Cuttoff (minThr)
      | else output is zero.
  In5 : Inport
  Constant : Constant  Value=quadModel.b
  Gain : Gain  Gain=quadModel.cr
  Minimum Throttle Cutoff : simulink/Logic and Bit Operations/Compare To Constant  relop=>=  const=quadModel.minThr  OutDataTypeStr=uint8
  Product : Product
  Sum1 : Sum  Inputs=++|
  Out5 : Outport
  wires:
  Minimum Throttle Cutoff/1 -> Product/2
  Product/1 -> Out5/1
  In5/1 -> Gain/1, Minimum Throttle Cutoff/1
  Gain/1 -> Sum1/2
  Sum1/1 -> Product/1
  Constant/1 -> Sum1/1

== system PC_Quadcopter_Simulation_Hexacopter_health/Position Controller/Motor Dynamics/Throttle To RPM Gain and Cutoff_3 ==
  note: minThr should be a quad.mat value
  note: This gain should be a quad.mat value
  note: This constant should be a quad.mat value
  note: Output equals linearly scaled RPM
      | for given throttle input if throttle input >=Throttle Cuttoff (minThr)
      | else output is zero.
  In5 : Inport
  Constant : Constant  Value=quadModel.b
  Gain : Gain  Gain=quadModel.cr
  Minimum Throttle Cutoff : simulink/Logic and Bit Operations/Compare To Constant  relop=>=  const=quadModel.minThr  OutDataTypeStr=uint8
  Product : Product
  Sum1 : Sum  Inputs=++|
  Out5 : Outport
  wires:
  Minimum Throttle Cutoff/1 -> Product/2
  Product/1 -> Out5/1
  In5/1 -> Gain/1, Minimum Throttle Cutoff/1
  Gain/1 -> Sum1/2
  Sum1/1 -> Product/1
  Constant/1 -> Sum1/1

== system PC_Quadcopter_Simulation_Hexacopter_health/Position Controller/Motor Dynamics/Throttle To RPM Gain and Cutoff_4 ==
  note: minThr should be a quad.mat value
  note: This gain should be a quad.mat value
  note: This constant should be a quad.mat value
  note: Output equals linearly scaled RPM
      | for given throttle input if throttle input >=Throttle Cuttoff (minThr)
      | else output is zero.
  In5 : Inport
  Constant : Constant  Value=quadModel.b
  Gain : Gain  Gain=quadModel.cr
  Minimum Throttle Cutoff : simulink/Logic and Bit Operations/Compare To Constant  relop=>=  const=quadModel.minThr  OutDataTypeStr=uint8
  Product : Product
  Sum1 : Sum  Inputs=++|
  Out5 : Outport
  wires:
  Minimum Throttle Cutoff/1 -> Product/2
  Product/1 -> Out5/1
  In5/1 -> Gain/1, Minimum Throttle Cutoff/1
  Gain/1 -> Sum1/2
  Sum1/1 -> Product/1
  Constant/1 -> Sum1/1

== system PC_Quadcopter_Simulation_Hexacopter_health/Position Controller/Motor Dynamics/Throttle To RPM Gain and Cutoff_5 ==
  note: minThr should be a quad.mat value
  note: This gain should be a quad.mat value
  note: This constant should be a quad.mat value
  note: Output equals linearly scaled RPM
      | for given throttle input if throttle input >=Throttle Cuttoff (minThr)
      | else output is zero.
  In5 : Inport
  Constant : Constant  Value=quadModel.b
  Gain : Gain  Gain=quadModel.cr
  Minimum Throttle Cutoff : simulink/Logic and Bit Operations/Compare To Constant  relop=>=  const=quadModel.minThr  OutDataTypeStr=uint8
  Product : Product
  Sum1 : Sum  Inputs=++|
  Out5 : Outport
  wires:
  Minimum Throttle Cutoff/1 -> Product/2
  Product/1 -> Out5/1
  In5/1 -> Gain/1, Minimum Throttle Cutoff/1
  Gain/1 -> Sum1/2
  Sum1/1 -> Product/1
  Constant/1 -> Sum1/1

== system PC_Quadcopter_Simulation_Hexacopter_health/Position Controller/Motor Dynamics/Throttle To RPM Gain and Cutoff_6 ==
  note: minThr should be a quad.mat value
  note: This gain should be a quad.mat value
  note: This constant should be a quad.mat value
  note: Output equals linearly scaled RPM
      | for given throttle input if throttle input >=Throttle Cuttoff (minThr)
      | else output is zero.
  In5 : Inport
  Constant : Constant  Value=quadModel.b
  Gain : Gain  Gain=quadModel.cr
  Minimum Throttle Cutoff : simulink/Logic and Bit Operations/Compare To Constant  relop=>=  const=quadModel.minThr  OutDataTypeStr=uint8
  Product : Product
  Sum1 : Sum  Inputs=++|
  Out5 : Outport
  wires:
  Minimum Throttle Cutoff/1 -> Product/2
  Product/1 -> Out5/1
  In5/1 -> Gain/1, Minimum Throttle Cutoff/1
  Gain/1 -> Sum1/2
  Sum1/1 -> Product/1
  Constant/1 -> Sum1/1

== matlab function PC_Quadcopter_Simulation_Hexacopter_health/Fault Diagnosis/Generate Residual/MATLAB Function - Generate Predicted Output ==
  data: xEstimated input; yPredicted output; u input
function yPredicted = generatePredictedOutput(xEstimated,u)

%   Copyright 2017 The MathWorks, Inc.

%#codegen

% Given state estimates at previous time (k-1) utilizing measurements up to
% (k-1), predict states at current step.
xPredicted = myStateTransitionFcn(xEstimated,u); % xhat[k|k-1]
% Generate output estimate, again without utilizing the measurement at
% current time.
yPredicted = myMeasurementFcn(xPredicted); % y[k|k-1]
end

== matlab function PC_Quadcopter_Simulation_Hexacopter_health/Hexacopter Control Mixing/MATLAB Function ==
  data: u input; y output
function y = fcn(u)
%% mixing matrix: PID correction to motors
m = 1.023;
g = 9.81;
ct = 1.4865e-07;
cr = 80.5840;
b = 976.2;
%% health state 6*1
h = u(5:10,1);
FDI = u(11,1);
% 
% A = [
%     -1/h(1,1) -1/h(1,1) -1/h(1,1) 1/h(1,1)
%     1/h(2,1) -1/h(2,1) 1/h(2,1) 1/h(2,1)
%     1/h(3,1) 0 -1/h(3,1) 1/h(3,1)
%     1/h(4,1) 1/h(4,1) 1/h(4,1) 1/h(4,1)
%     -1/h(5,1) 1/h(5,1) -1/h(5,1) 1/h(5,1)
%     -1/h(6,1) 0 1/h(6,1) 1/h(6,1)
%     ];

A = [
    -1 -1 -1 1
    1 -1 1 1
    1 0 -1 1
    1 1 1 1
    -1 1 -1 1
    -1 0 1 1
    ];

%% 고장을 고려한 mixing 변화
if FDI==1 | FDI==4
h(1,1)=0;
h(2,1)=1;
h(3,1)=1;
h(4,1)=0;
h(5,1)=1;
h(6,1)=1;

A = [
    -1 -1 -1 1
    1 -1 1 1
    1 0 -1 1
    1 1 1 1
    -1 1 -1 1
    -1 0 1 1
    ];

elseif FDI==2 | FDI==5
h(1,1)=1;
h(2,1)=0;
h(3,1)=1;
h(4,1)=1;
h(5,1)=0;
h(6,1)=1;

A = [
    -1 -1 -1 1
    1 -1 1 1
    1 0 -1 1
    1 1 1 1
    -1 1 -1 1
    -1 0 1 1
    ];

elseif FDI==3 | FDI==6
h(1,1)=1;
h(2,1)=1;
h(3,1)=0;
h(4,1)=1;
h(5,1)=1;
h(6,1)=0;
% 
A = [
    -1 -1 -1 1
    1 -1 1 1
    1 0 -1 1
    1 1 1 1
    -1 1 -1 1
    -1 0 1 1
    ];

end
for i=1:6
    A(i,:) = h(i)*A(i,:);
end

%% 고장을 고려한 건강한 모터의 추력 증가
% A = sqrt(6/sum(h))*A;


y = A*( u(1:4,:) )
% y = A*( u(1:4,:) ) + (sqrt(m*g/sum(h)/ct)-b)/cr ...
%     - (sqrt(m*g/6/ct)-b)/cr ;

== matlab function PC_Quadcopter_Simulation_Hexacopter_health/Fault Diagnosis/MATLAB Function ==
  data: p input; y output; q input; r input; a_z input; Z input; h input; t input
function y = FDI(p,q,r,a_z,Z,h,t)
% th = 0.04;
p_th = 0.03;
q_th = 0.07;
r_th = 0.015;
% z_th = 0.001;
%  & a_z<-z_th
y=0;

while y==0
    if  Z>0 & p>p_th & q>q_th & r>r_th & h(1) < 0.88 | t>0.2 & h(1) < 0.6
        y=1;
    elseif Z>0 & p<-p_th & q>q_th & r<-r_th & h(2) < 0.88 | t>0.2 & h(2) < 0.6
        y=2;
    elseif Z>0 & p<-p_th & -q_th<q & q<q_th & r>r_th & h(3) < 0.88 | t>0.2 & h(3) < 0.6
        y=3;
    elseif Z>0 & p<-p_th & q<-q_th & r<-r_th & h(4) < 0.88 | t>0.2 & h(4) < 0.6
        y=4;
    elseif Z>0 & p>p_th & q<-q_th & r>r_th & h(5) < 0.88 | t>0.2 & h(5) < 0.6
        y=5;
%     elseif Z>0 & p>p_th & -q_th<q & q<q_th & r<-r_th  & h(6) < 0.88 | t>0.2 & h(6) < 0.6
%         y=6;
    end
    break
end            
end

== matlab function PC_Quadcopter_Simulation_Hexacopter_health/Fault Diagnosis/MATLAB Function1 ==
  data: R1 input; y output; R2 input; R3 input; R4 input; R5 input; R6 input; Z input; h input; t input
function y = FDI(R1,R2,R3,R4,R5,R6,Z,h,t)
% th = 0.04;
RPM_th = 1000;

y=0;

while y==0
    if  Z>0 & t>0.5 & R1>RPM_th & h(1) < 0.6 
%         | t>0.2 & h(1) < 0.55
        y=1;
    elseif Z>0 & t>0.5 & R2>RPM_th & h(2) < 0.6 
        y=2;
    elseif Z>0 & t>0.5 & R3>RPM_th & h(3) < 0.6 
%         | t>0.5 & h(3) < 0.6
        y=3;
    elseif Z>0 & t>0.5 & R4>RPM_th & h(4) < 0.6 
        y=4;
    elseif Z>0 & t>0.5 & R5>RPM_th & h(5) < 0.6 
        y=5;
%     elseif Z>0 & t>0.5 & R6>RPM_th & h(6) < 0.6 | Z>0 & t>0.5 & R6<-RPM_th & h(6) < 0.6
%         y=6;
    end
    break
end            
end

== matlab function PC_Quadcopter_Simulation_Hexacopter_health/Position Controller/Hexacopter Control Mixing/MATLAB Function ==
  data: u input; y output
function y = fcn(u)
%% mixing matrix: PID correction to motors
m = 1.023;
g = 9.81;
ct = 1.4865e-07;
cr = 80.5840;
b = 976.2;
%% health state 6*1
h = u(5:10,1);
FDI = u(11,1);
% 
% A = [
%     -1/h(1,1) -1/h(1,1) -1/h(1,1) 1/h(1,1)
%     1/h(2,1) -1/h(2,1) 1/h(2,1) 1/h(2,1)
%     1/h(3,1) 0 -1/h(3,1) 1/h(3,1)
%     1/h(4,1) 1/h(4,1) 1/h(4,1) 1/h(4,1)
%     -1/h(5,1) 1/h(5,1) -1/h(5,1) 1/h(5,1)
%     -1/h(6,1) 0 1/h(6,1) 1/h(6,1)
%     ];

A = [
    -1 -1 -1 1
    1 -1 1 1
    1 0 -1 1
    1 1 1 1
    -1 1 -1 1
    -1 0 1 1
    ];

%% 고장을 고려한 mixing 변화
if FDI==1 | FDI==4
h(1,1)=0;
h(2,1)=1;
h(3,1)=1;
h(4,1)=0;
h(5,1)=1;
h(6,1)=1;

A = [
    -1 -1 -1 1
    1 -1 1 1
    1 0 -1 1
    1 1 1 1
    -1 1 -1 1
    -1 0 1 1
    ];

elseif FDI==2 | FDI==5
h(1,1)=1;
h(2,1)=0;
h(3,1)=1;
h(4,1)=1;
h(5,1)=0;
h(6,1)=1;

A = [
    -1 -1 -1 1
    1 -1 1 1
    1 0 -1 1
    1 1 1 1
    -1 1 -1 1
    -1 0 1 1
    ];

elseif FDI==3 | FDI==6
h(1,1)=1;
h(2,1)=1;
h(3,1)=0;
h(4,1)=1;
h(5,1)=1;
h(6,1)=0;
% 
A = [
    -1 -1 -1 1
    1 -1 1 1
    1 0 -1 1
    1 1 1 1
    -1 1 -1 1
    -1 0 1 1
    ];

end
for i=1:6
    A(i,:) = h(i)*A(i,:);
end

%% 고장을 고려한 건강한 모터의 추력 증가
% A = sqrt(6/sum(h))*A;


y = A*( u(1:4,:) )
% y = A*( u(1:4,:) ) + (sqrt(m*g/sum(h)/ct)-b)/cr ...
%     - (sqrt(m*g/6/ct)-b)/cr ;
